simulink model "SF045A_HwAgSysArbn"  (R2013b)
settings: Solver=FixedStepDiscrete  SolverMode=SingleTasking  StartTime=0.0  StopTime=1  FixedStep=.002  RelTol=1e-3
values from neighbouring files (symbols this model uses):
  ARCHGLBPRM_2MILLISEC_SEC_F32 = DataDict.Constant    [SF045A_HwAgSysArbn_DataDict.m]
  ARCHGLBPRM_FLOATZEROTHD_ULS_F32 = DataDict.Constant    [SF045A_HwAgSysArbn_DataDict.m]
  ARCHGLBPRM_PIOVER180_ULS_F32 = DataDict.Constant    [SF045A_HwAgSysArbn_DataDict.m]
  CNVSECTOCNT_ULS_U32 = DataDict.Constant    [SF045A_HwAgSysArbn_DataDict.m]
  CNVTOMILLISEC_MILLISECPERCNT_F32 = DataDict.Constant    [SF045A_HwAgSysArbn_DataDict.m]
  FltInj_f32 = DataDict.Client    [SF045A_HwAgSysArbn_DataDict.m]
  FLTINJ_HWAGSYSARBN_HWAG = DataDict.Constant    [SF045A_HwAgSysArbn_DataDict.m]
  FLTINJ_HWAGSYSARBN_SERLCOMHWAG = DataDict.Constant    [SF045A_HwAgSysArbn_DataDict.m]
  HwAgCorrlnFlt = DataDict.NTC    [SF045A_HwAgSysArbn_DataDict.m]
  HwAgSnsrlsThdExcdd = DataDict.NTC    [SF045A_HwAgSysArbn_DataDict.m]
  HwAgSysArbnHwAgConf1Snsr = DataDict.Calibration    [SF045A_HwAgSysArbn_DataDict.m]
  HwAgSysArbnHwAgConf2Snsr = DataDict.Calibration    [SF045A_HwAgSysArbn_DataDict.m]
  HwAgSysArbnHwAgConfNoSnsr = DataDict.Calibration    [SF045A_HwAgSysArbn_DataDict.m]
  HwAgSysArbnHwAgCorrdCorrlnThd = DataDict.Calibration    [SF045A_HwAgSysArbn_DataDict.m]
  HwAgSysArbnHwAgCorrlnFailDebStep = DataDict.Calibration    [SF045A_HwAgSysArbn_DataDict.m]
  HwAgSysArbnHwAgCorrlnPassDebStep = DataDict.Calibration    [SF045A_HwAgSysArbn_DataDict.m]
  HwAgSysArbnHwAgCorrlnRng = DataDict.Calibration    [SF045A_HwAgSysArbn_DataDict.m]
  HwAgSysArbnHwAgSlewRate = DataDict.Calibration    [SF045A_HwAgSysArbn_DataDict.m]
  HwAgSysArbnHwAgSnsrlsCorrlnThd = DataDict.Calibration    [SF045A_HwAgSysArbn_DataDict.m]
  HwAgSysArbnHwAgSnsrlsKineThd = DataDict.Calibration    [SF045A_HwAgSysArbn_DataDict.m]
  HwAgSysArbnHwAgToMotAgCorrlnElpdTiLim = DataDict.Calibration    [SF045A_HwAgSysArbn_DataDict.m]
  HwAgSysArbnSerlComHwAgCorrdConf = DataDict.Calibration    [SF045A_HwAgSysArbn_DataDict.m]
  HwAgSysArbnSerlComHwAgSnsrlsConf = DataDict.Calibration    [SF045A_HwAgSysArbn_DataDict.m]
  HwAgSysArbnSlewRateTmr = DataDict.Calibration    [SF045A_HwAgSysArbn_DataDict.m]
  HWAGTHD_ULS_FLOAT32 = DataDict.Constant    [SF045A_HwAgSysArbn_DataDict.m]
  INVLDSRC_CNT_S08 = DataDict.Constant    [SF045A_HwAgSysArbn_DataDict.m]
  LRGSLEW_HWDEGPERSEC_F32 = DataDict.Constant    [SF045A_HwAgSysArbn_DataDict.m]
  NODEBSTEP_CNT_U16 = DataDict.Constant    [SF045A_HwAgSysArbn_DataDict.m]
  SLEWINPROGS_CNT_LGC = DataDict.Constant    [SF045A_HwAgSysArbn_DataDict.m]
  SLEWNOTINPROGS_CNT_LGC = DataDict.Constant    [SF045A_HwAgSysArbn_DataDict.m]
  SNSRDATASRCSELD_CNT_S08 = DataDict.Constant    [SF045A_HwAgSysArbn_DataDict.m]
  SNSRLSDATASRCSELD_CNT_S08 = DataDict.Constant    [SF045A_HwAgSysArbn_DataDict.m]
  SysGlbPrmSysKineRat = DataDict.ImprtdCal    [SF045A_HwAgSysArbn_DataDict.m]
  SysGlbPrmTorsBarStfn = DataDict.ImprtdCal    [SF045A_HwAgSysArbn_DataDict.m]
  ZEROTMR_MILLISEC_F32 = DataDict.Constant    [SF045A_HwAgSysArbn_DataDict.m]
undefined symbols (not defined in the file or in its folder): NtcSts1
libraries: NxtrLim x11, simulink x6, NxtrAbslt x6, Fil x3, autosarlib x2
(part 3 of 6)

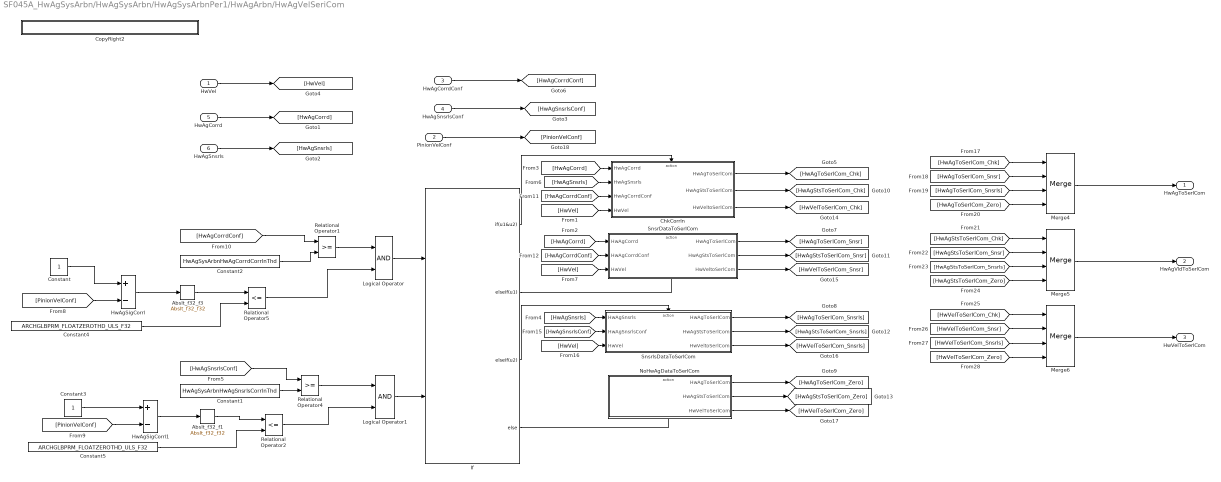
== system SF045A_HwAgSysArbn/HwAgSysArbn/HwAgSysArbnPer1/HwAgArbn/HwAgVelSeriCom ==
  HwVel : Inport
  PinionVelConf : Inport  Port=2
  HwAgCorrdConf : Inport  Port=3
  HwAgSnsrlsConf : Inport  Port=4
  HwAgCorrd : Inport  Port=5
  HwAgSnsrls : Inport  Port=6
  Abslt_f32_f1 : NxtrAbslt/Abslt_f32_f32  RequirementInfo={} %GIDa_b8a4dc3f_585f_4398_a9f9_8fc984254714  SFunctionSpec=single y1 = Abslt_f32_f32(single u1)
      settings: AttributesFormatString=%<Name>
  Abslt_f32_f3 : NxtrAbslt/Abslt_f32_f32  RequirementInfo={} %GIDa_7c7c182e_46fe_47af_9f86_60131a6a4daf  SFunctionSpec=single y1 = Abslt_f32_f32(single u1)
      settings: AttributesFormatString=%<Name>
  ChkCorrln : Subsystem  RequirementInfo="{'linktype_rmi_doors' '00012ce0 (/E-STEER Core/SubSystem Specifications/Application Functions - EA4/SF045A Handwheel Angle System Arbitration)' '#SF045A_104' 'true' 'REQ:  SF045A_104' '' ; 'linktype_rmi_doors' '00012ce0 (/E-STEER Core/SubSystem Specifications/Application Functions - EA4/SF045A Handwheel Angle System Arbitration)' '#SF045A_105' 'true' 'REQ:  SF045A_105' '' ; 'linktype_rmi_doors' '00012ce0 (/E-STEER Core/SubSystem Specifications/Application Functions - EA4/SF045A Handwheel Angle System Arbitration)' '#SF045A_141' 'true' 'REQ:  SF045A_141' '' } %GIDa_01d8e59b_3b0f_4a53_93ac_fe398fdd2570"  TreatAsAtomicUnit=on
  Constant : Constant  OutDataTypeStr=single
      settings: AttributesFormatString=%<OutDataTypeStr>
  Constant1 : Constant  RequirementInfo={} %GIDa_66b39656_3ea7_4f1f_ba8a_04f304451550  Value=HwAgSysArbnHwAgSnsrlsCorrlnThd  OutDataTypeStr=single
  Constant2 : Constant  RequirementInfo={} %GIDa_c72f589f_146e_4a47_a32d_f0a439dbf3d4  Value=HwAgSysArbnHwAgCorrdCorrlnThd  OutDataTypeStr=single
  Constant3 : Constant  OutDataTypeStr=single
      settings: AttributesFormatString=%<OutDataTypeStr>
  Constant4 : Constant  RequirementInfo={} %GIDa_2ba92f60_c072_4a0f_905b_124fe50057e6  Value=ARCHGLBPRM_FLOATZEROTHD_ULS_F32
  Constant5 : Constant  RequirementInfo={} %GIDa_95ac923c_5133_4b3b_b37a_4089be04068f  Value=ARCHGLBPRM_FLOATZEROTHD_ULS_F32
  CopyRight2 : Subsystem  Description=|  mask(Copyright Information){none=on}
      | Copyright info block.                                               
      |                                                                     
      | Place copyright information at the top of every subsystem in design.
      mask prompts: none "No parameters"
      mask help: Place copyright information at the top of every subsystem in design.
      mask Display:
      | NxtrConf = 'Nexteer Confidential';
      | 
      | sys = bdroot; %handle for the current model ("system")
      | first = get_param(sys,'Created');
      | first = first(end-3:end);  %year is last four digits
      | 
      | last = get_param(sys,'LastModifiedDate');
      | if isempty(last)
      |     last = datestr(now,'yyyy');
      | else
      |     last = last(end-3:end);
      | end
      | 
      | if strcmp(first,last)
      |     fprintf('%s -- Copyright %s Nexteer',NxtrConf,first)
      | else
      |     fprintf('%s -- %s%s- %s Nexteer',NxtrConf,char(169),first,last)
      | end
  HwAgSigCorrl : Sum  RequirementInfo="{'linktype_rmi_doors' '00012ce0 (/E-STEER Core/SubSystem Specifications/Application Functions - EA4/SF045A Handwheel Angle System Arbitration)' '#SF045A_105' 'true' 'REQ:  SF045A_105' '' } %GIDa_d7192d38_61ab_4c5a_8ed7_a2ef9f470f72"  Inputs=+-
  HwAgSigCorrl1 : Sum  RequirementInfo="{'linktype_rmi_doors' '00012ce0 (/E-STEER Core/SubSystem Specifications/Application Functions - EA4/SF045A Handwheel Angle System Arbitration)' '#SF045A_105' 'true' 'REQ:  SF045A_105' '' } %GIDa_e3eac1c3_2ea3_4330_ab07_f70996d04291"  Inputs=+-
  If : If  RequirementInfo="{'linktype_rmi_doors' '00012ce0 (/E-STEER Core/SubSystem Specifications/Application Functions - EA4/SF045A Handwheel Angle System Arbitration)' '#SF045A_85' 'true' 'REQ:  SF045A_85' '' ; 'linktype_rmi_doors' '00012ce0 (/E-STEER Core/SubSystem Specifications/Application Functions - EA4/SF045A Handwheel Angle System Arbitration)' '#SF045A_86' 'true' 'REQ:  SF045A_86' '' ; 'linktype_rmi_doors' '00012ce0 (/E-STEER Core/SubSystem Specifications/Application Functions - EA4/SF045A Handwheel Angle System Arbitration)' '#SF045A_90' 'true' 'REQ:  SF045A_90' '' ; 'linktype_rmi_doors' '00012ce0 (/E-STEER Core/SubSystem Specifications/Application Functions - EA4/SF045A Handwheel Angle System Arbitration)' '#SF045A_141' 'true' 'REQ:  SF045A_141' '' } %GIDa_16295e6d_604c_4ea2_8003_45c4a31ea523"  NumInputs=2  IfExpression=u1&u2  ElseIfExpressions=u1, u2
  Logical Operator : Logic  RequirementInfo="{'linktype_rmi_doors' '00012ce0 (/E-STEER Core/SubSystem Specifications/Application Functions - EA4/SF045A Handwheel Angle System Arbitration)' '#SF045A_104' 'true' 'REQ:  SF045A_104' '' ; 'linktype_rmi_doors' '00012ce0 (/E-STEER Core/SubSystem Specifications/Application Functions - EA4/SF045A Handwheel Angle System Arbitration)' '#SF045A_85' 'true' 'REQ:  SF045A_85' '' } %GIDa_dce261ed_e3ab_4b88_85ed_bb93f578dcbd"  AllPortsSameDT=off  OutDataTypeStr=boolean
  Logical Operator1 : Logic  RequirementInfo="{'linktype_rmi_doors' '00012ce0 (/E-STEER Core/SubSystem Specifications/Application Functions - EA4/SF045A Handwheel Angle System Arbitration)' '#SF045A_104' 'true' 'REQ:  SF045A_104' '' ; 'linktype_rmi_doors' '00012ce0 (/E-STEER Core/SubSystem Specifications/Application Functions - EA4/SF045A Handwheel Angle System Arbitration)' '#SF045A_86' 'true' 'REQ:  SF045A_86' '' } %GIDa_f647724d_ceef_4875_8752_3049c96c44e3"  AllPortsSameDT=off  OutDataTypeStr=boolean
  Merge4 : Merge  RequirementInfo="{'linktype_rmi_doors' '00012ce0 (/E-STEER Core/SubSystem Specifications/Application Functions - EA4/SF045A Handwheel Angle System Arbitration)' '#SF045A_85' 'true' 'REQ:  SF045A_85' '' ; 'linktype_rmi_doors' '00012ce0 (/E-STEER Core/SubSystem Specifications/Application Functions - EA4/SF045A Handwheel Angle System Arbitration)' '#SF045A_86' 'true' 'REQ:  SF045A_86' '' ; 'linktype_rmi_doors' '00012ce0 (/E-STEER Core/SubSystem Specifications/Application Functions - EA4/SF045A Handwheel Angle System Arbitration)' '#SF045A_141' 'true' 'REQ:  SF045A_141' '' ; 'linktype_rmi_doors' '00012ce0 (/E-STEER Core/SubSystem Specifications/Application Functions - EA4/SF045A Handwheel Angle System Arbitration)' '#SF045A_90' 'true' 'REQ:  SF045A_90' '' } %GIDa_63d2fbfa_6b1d_45be_95e0_66958795916e"  Inputs=4
  Merge5 : Merge  RequirementInfo="{'linktype_rmi_doors' '00012ce0 (/E-STEER Core/SubSystem Specifications/Application Functions - EA4/SF045A Handwheel Angle System Arbitration)' '#SF045A_85' 'true' 'REQ:  SF045A_85' '' ; 'linktype_rmi_doors' '00012ce0 (/E-STEER Core/SubSystem Specifications/Application Functions - EA4/SF045A Handwheel Angle System Arbitration)' '#SF045A_86' 'true' 'REQ:  SF045A_86' '' ; 'linktype_rmi_doors' '00012ce0 (/E-STEER Core/SubSystem Specifications/Application Functions - EA4/SF045A Handwheel Angle System Arbitration)' '#SF045A_141' 'true' 'REQ:  SF045A_141' '' ; 'linktype_rmi_doors' '00012ce0 (/E-STEER Core/SubSystem Specifications/Application Functions - EA4/SF045A Handwheel Angle System Arbitration)' '#SF045A_90' 'true' 'REQ:  SF045A_90' '' } %GIDa_9d75f2ca_ac61_4030_ae3e_b2f03a9d1071"  Inputs=4
  Merge6 : Merge  RequirementInfo="{'linktype_rmi_doors' '00012ce0 (/E-STEER Core/SubSystem Specifications/Application Functions - EA4/SF045A Handwheel Angle System Arbitration)' '#SF045A_85' 'true' 'REQ:  SF045A_85' '' ; 'linktype_rmi_doors' '00012ce0 (/E-STEER Core/SubSystem Specifications/Application Functions - EA4/SF045A Handwheel Angle System Arbitration)' '#SF045A_86' 'true' 'REQ:  SF045A_86' '' ; 'linktype_rmi_doors' '00012ce0 (/E-STEER Core/SubSystem Specifications/Application Functions - EA4/SF045A Handwheel Angle System Arbitration)' '#SF045A_141' 'true' 'REQ:  SF045A_141' '' ; 'linktype_rmi_doors' '00012ce0 (/E-STEER Core/SubSystem Specifications/Application Functions - EA4/SF045A Handwheel Angle System Arbitration)' '#SF045A_90' 'true' 'REQ:  SF045A_90' '' } %GIDa_8dbea807_2d0b_4205_9136_c887d8e00053"  Inputs=4
  NoHwAgDataToSerlCom : Subsystem  RequirementInfo="{'linktype_rmi_doors' '00012ce0 (/E-STEER Core/SubSystem Specifications/Application Functions - EA4/SF045A Handwheel Angle System Arbitration)' '#SF045A_90' 'true' 'REQ:  SF045A_90' '' } %GIDa_e15506f9_dc76_46a3_abc9_05bc78f3206f"  TreatAsAtomicUnit=on
  Relational Operator1 : RelationalOperator  RequirementInfo="{'linktype_rmi_doors' '00012ce0 (/E-STEER Core/SubSystem Specifications/Application Functions - EA4/SF045A Handwheel Angle System Arbitration)' '#SF045A_104' 'true' 'REQ:  SF045A_104' '' ; 'linktype_rmi_doors' '00012ce0 (/E-STEER Core/SubSystem Specifications/Application Functions - EA4/SF045A Handwheel Angle System Arbitration)' '#SF045A_85' 'true' 'REQ:  SF045A_85' '' } %GIDa_a51aeb99_538c_4fd9_86fe_31ab29bb7151"  OutDataTypeStr=boolean
  Relational Operator2 : RelationalOperator  RequirementInfo="{'linktype_rmi_doors' '00012ce0 (/E-STEER Core/SubSystem Specifications/Application Functions - EA4/SF045A Handwheel Angle System Arbitration)' '#SF045A_104' 'true' 'REQ:  SF045A_104' '' ; 'linktype_rmi_doors' '00012ce0 (/E-STEER Core/SubSystem Specifications/Application Functions - EA4/SF045A Handwheel Angle System Arbitration)' '#SF045A_85' 'true' 'REQ:  SF045A_85' '' } %GIDa_fbe37bb0_44f1_4683_abd9_0356a5e60375"  Operator=<=  OutDataTypeStr=boolean
  Relational Operator4 : RelationalOperator  RequirementInfo="{'linktype_rmi_doors' '00012ce0 (/E-STEER Core/SubSystem Specifications/Application Functions - EA4/SF045A Handwheel Angle System Arbitration)' '#SF045A_104' 'true' 'REQ:  SF045A_104' '' ; 'linktype_rmi_doors' '00012ce0 (/E-STEER Core/SubSystem Specifications/Application Functions - EA4/SF045A Handwheel Angle System Arbitration)' '#SF045A_86' 'true' 'REQ:  SF045A_86' '' } %GIDa_5ff63e87_12bf_4da7_987b_69d09a6b50ad"  OutDataTypeStr=boolean
  Relational Operator5 : RelationalOperator  RequirementInfo="{'linktype_rmi_doors' '00012ce0 (/E-STEER Core/SubSystem Specifications/Application Functions - EA4/SF045A Handwheel Angle System Arbitration)' '#SF045A_104' 'true' 'REQ:  SF045A_104' '' ; 'linktype_rmi_doors' '00012ce0 (/E-STEER Core/SubSystem Specifications/Application Functions - EA4/SF045A Handwheel Angle System Arbitration)' '#SF045A_85' 'true' 'REQ:  SF045A_85' '' } %GIDa_f786c2da_ebce_4ccd_8e6f_5c0e8e3ac68c"  Operator=<=  OutDataTypeStr=boolean
  SnsrDataToSerlCom : Subsystem  RequirementInfo="{'linktype_rmi_doors' '00012ce0 (/E-STEER Core/SubSystem Specifications/Application Functions - EA4/SF045A Handwheel Angle System Arbitration)' '#SF045A_85' 'true' 'REQ:  SF045A_85' '' } %GIDa_75d9779f_c388_4d50_b433_ec26c71a85aa"  TreatAsAtomicUnit=on
  SnsrlsDataToSerlCom : Subsystem  RequirementInfo="{'linktype_rmi_doors' '00012ce0 (/E-STEER Core/SubSystem Specifications/Application Functions - EA4/SF045A Handwheel Angle System Arbitration)' '#SF045A_86' 'true' 'REQ:  SF045A_86' '' ; 'linktype_rmi_doors' '00012ce0 (/E-STEER Core/SubSystem Specifications/Application Functions - EA4/SF045A Handwheel Angle System Arbitration)' '#SF045A_126' 'true' 'REQ:  SF045A_126' '' ; 'linktype_rmi_doors' '00012ce0 (/E-STEER Core/SubSystem Specifications/Application Functions - EA4/SF045A Handwheel Angle System Arbitration)' '#SF045A_124' 'true' 'REQ:  SF045A_124' '' ; 'linktype_rmi_doors' '00012ce0 (/E-STEER Core/SubSystem Specifications/Application Functions - EA4/SF045A Handwheel Angle System Arbitration)' '#SF045A_88' 'true' 'REQ:  SF045A_88' '' } %GIDa_d8bafae9_7cb5_4a99_9cbb_12d18e69b352"  TreatAsAtomicUnit=on
  HwAgToSerlCom : Outport
  HwAgVldToSerlCom : Outport  Port=2
  HwVelToSerlCom : Outport  Port=3
  wires:
  [HwAgSnsrls] -> ChkCorrln/2(HwAgSnsrls)
  [HwAgCorrdConf] -> Relational Operator1/1
  Constant2/1 -> Relational Operator1/2
  [HwAgSnsrlsConf] -> Relational Operator4/1
  Constant1/1 -> Relational Operator4/2
  If/1 -> ChkCorrln/Action
  [HwAgCorrd] -> ChkCorrln/1(HwAgCorrd)
  If/2 -> SnsrDataToSerlCom/Action
  [HwAgCorrd] -> SnsrDataToSerlCom/1(HwAgCorrd)
  [HwAgSnsrls] -> SnsrlsDataToSerlCom/1(HwAgSnsrls)
  If/3 -> SnsrlsDataToSerlCom/Action
  If/4 -> NoHwAgDataToSerlCom/Action
  [HwAgCorrdConf] -> ChkCorrln/3(HwAgCorrdConf)
  [HwAgCorrdConf] -> SnsrDataToSerlCom/2(HwAgCorrdConf)
  [HwAgSnsrlsConf] -> SnsrlsDataToSerlCom/2(HwAgSnsrlsConf)
  Merge4/1 -> HwAgToSerlCom/1
  Relational Operator1/1 -> Logical Operator/1
  Logical Operator/1 -> If/1
  Logical Operator1/1 -> If/2
  Relational Operator4/1 -> Logical Operator1/1
  [HwVel] -> ChkCorrln/4(HwVel)
  [HwVel] -> SnsrDataToSerlCom/3(HwVel)
  [HwVel] -> SnsrlsDataToSerlCom/3(HwVel)
  ChkCorrln/1(HwAgToSerlCom) -> [HwAgToSerlCom_Chk]
  SnsrDataToSerlCom/1(HwAgToSerlCom) -> [HwAgToSerlCom_Snsr]
  SnsrlsDataToSerlCom/1(HwAgToSerlCom) -> [HwAgToSerlCom_Snsrls]
  NoHwAgDataToSerlCom/1(HwAgToSerlCom) -> [HwAgToSerlCom_Zero]
  [HwAgToSerlCom_Chk] -> Merge4/1
  [HwAgToSerlCom_Snsr] -> Merge4/2
  [HwAgToSerlCom_Snsrls] -> Merge4/3
  [HwAgToSerlCom_Zero] -> Merge4/4
  ChkCorrln/2(HwAgStsToSerlCom) -> [HwAgStsToSerlCom_Chk]
  ChkCorrln/3(HwVeltoSerlCom) -> [HwVelToSerlCom_Chk]
  SnsrDataToSerlCom/2(HwAgStsToSerlCom) -> [HwAgStsToSerlCom_Snsr]
  SnsrDataToSerlCom/3(HwVeltoSerlCom) -> [HwVelToSerlCom_Snsr]
  SnsrlsDataToSerlCom/2(HwAgStsToSerlCom) -> [HwAgStsToSerlCom_Snsrls]
  SnsrlsDataToSerlCom/3(HwVeltoSerlCom) -> [HwVelToSerlCom_Snsrls]
  NoHwAgDataToSerlCom/2(HwAgStsToSerlCom) -> [HwAgStsToSerlCom_Zero]
  NoHwAgDataToSerlCom/3(HwVelToSerlCom) -> [HwVelToSerlCom_Zero]
  [HwAgStsToSerlCom_Chk] -> Merge5/1
  [HwAgStsToSerlCom_Snsr] -> Merge5/2
  [HwAgStsToSerlCom_Snsrls] -> Merge5/3
  [HwAgStsToSerlCom_Zero] -> Merge5/4
  [HwVelToSerlCom_Chk] -> Merge6/1
  [HwVelToSerlCom_Snsr] -> Merge6/2
  [HwVelToSerlCom_Snsrls] -> Merge6/3
  [HwVelToSerlCom_Zero] -> Merge6/4
  Merge6/1 -> HwVelToSerlCom/1
  HwVel/1 -> [HwVel]
  HwAgCorrdConf/1 -> [HwAgCorrdConf]
  HwAgSnsrlsConf/1 -> [HwAgSnsrlsConf]
  HwAgCorrd/1 -> [HwAgCorrd]
  HwAgSnsrls/1 -> [HwAgSnsrls]
  Merge5/1 -> HwAgVldToSerlCom/1
  PinionVelConf/1 -> [PinionVelConf]
  HwAgSigCorrl/1 -> Abslt_f32_f3/1
  Constant4/1 -> Relational Operator5/2
  Relational Operator5/1 -> Logical Operator/2
  Constant/1 -> HwAgSigCorrl/1
  [PinionVelConf] -> HwAgSigCorrl/2
  Abslt_f32_f3/1 -> Relational Operator5/1
  HwAgSigCorrl1/1 -> Abslt_f32_f1/1
  Constant5/1 -> Relational Operator2/2
  Constant3/1 -> HwAgSigCorrl1/1
  [PinionVelConf] -> HwAgSigCorrl1/2
  Abslt_f32_f1/1 -> Relational Operator2/1
  Relational Operator2/1 -> Logical Operator1/2

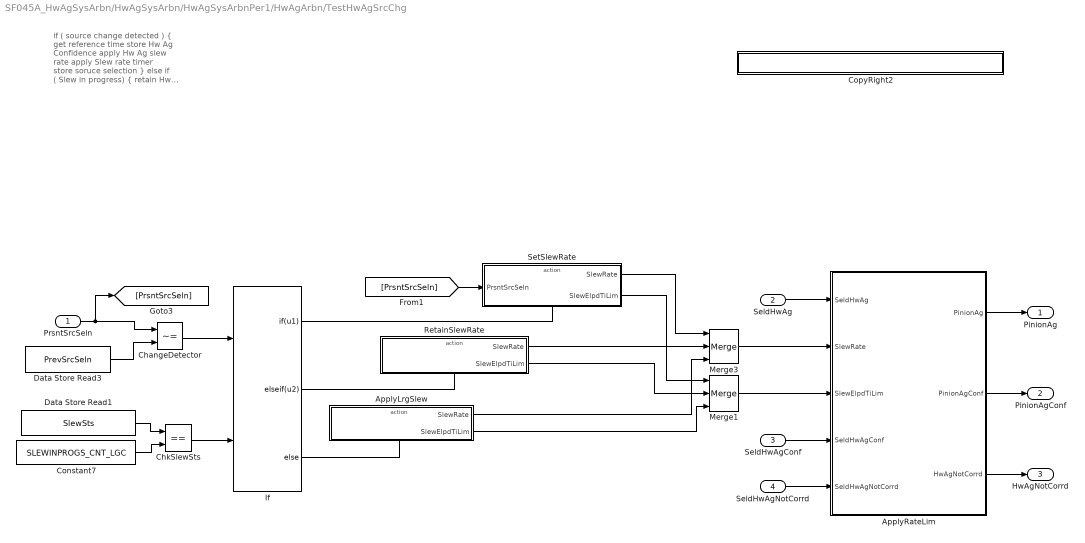
== system SF045A_HwAgSysArbn/HwAgSysArbn/HwAgSysArbnPer1/HwAgArbn/TestHwAgSrcChg ==
  note: if ( source change detected )
      | 	{
      |       get reference time
      |       store Hw Ag Confidence
      |       apply Hw Ag slew rate
      |       apply Slew rate timer
      |       store soruce selection
      | 	 }
      | else if ( Slew in progress)
      |      {
      |       retain Hw Ag slew rate
      |       retain Slew rate timer
      |       }
      |  else
      |    {
      |      apply large slew rate
      |      apply zero timer
      |     }
  PrsntSrcSeln : Inport
  SeldHwAg : Inport  Port=2
  SeldHwAgConf : Inport  Port=3
  SeldHwAgNotCorrd : Inport  Port=4
  ApplyLrgSlew : Subsystem  RequirementInfo="{'linktype_rmi_doors' '00012ce0 (/E-STEER Core/SubSystem Specifications/Application Functions - EA4/SF045A Handwheel Angle System Arbitration)' '#SF045A_77' 'true' 'REQ:  SF045A_77' '' ; 'linktype_rmi_doors' '00012ce0 (/E-STEER Core/SubSystem Specifications/Application Functions - EA4/SF045A Handwheel Angle System Arbitration)' '#SF045A_78' 'true' 'REQ:  SF045A_78' '' ; 'linktype_rmi_doors' '00012ce0 (/E-STEER Core/SubSystem Specifications/Application Functions - EA4/SF045A Handwheel Angle System Arbitration)' '#SF045A_79' 'true' 'REQ:  SF045A_79' '' } %GIDa_e44356f8_ec38_43bf_a50a_7696017339bb"  TreatAsAtomicUnit=on
  ApplyRateLim : Subsystem  RequirementInfo="{'linktype_rmi_doors' '00012ce0 (/E-STEER Core/SubSystem Specifications/Application Functions - EA4/SF045A Handwheel Angle System Arbitration)' '#SF045A_77' 'true' 'REQ:  SF045A_77' '' ; 'linktype_rmi_doors' '00012ce0 (/E-STEER Core/SubSystem Specifications/Application Functions - EA4/SF045A Handwheel Angle System Arbitration)' '#SF045A_78' 'true' 'REQ:  SF045A_78' '' ; 'linktype_rmi_doors' '00012ce0 (/E-STEER Core/SubSystem Specifications/Application Functions - EA4/SF045A Handwheel Angle System Arbitration)' '#SF045A_79' 'true' 'REQ:  SF045A_79' '' } %GIDa_f1478672_2f89_4aac_bacc_fec9bee029da"
  ChangeDetector : RelationalOperator  RequirementInfo="{'linktype_rmi_doors' '00012ce0 (/E-STEER Core/SubSystem Specifications/Application Functions - EA4/SF045A Handwheel Angle System Arbitration)' '#SF045A_77' 'true' 'REQ:  SF045A_77' '' ; 'linktype_rmi_doors' '00012ce0 (/E-STEER Core/SubSystem Specifications/Application Functions - EA4/SF045A Handwheel Angle System Arbitration)' '#SF045A_78' 'true' 'REQ:  SF045A_78' '' ; 'linktype_rmi_doors' '00012ce0 (/E-STEER Core/SubSystem Specifications/Application Functions - EA4/SF045A Handwheel Angle System Arbitration)' '#SF045A_79' 'true' 'REQ:  SF045A_79' '' } %GIDa_8b7e8362_f8ac_4ce7_bdd9_53ebc347e7a4"  Operator=~=  OutDataTypeStr=boolean
  ChkSlewSts : RelationalOperator  RequirementInfo="{'linktype_rmi_doors' '00012ce0 (/E-STEER Core/SubSystem Specifications/Application Functions - EA4/SF045A Handwheel Angle System Arbitration)' '#SF045A_77' 'true' 'REQ:  SF045A_77' '' ; 'linktype_rmi_doors' '00012ce0 (/E-STEER Core/SubSystem Specifications/Application Functions - EA4/SF045A Handwheel Angle System Arbitration)' '#SF045A_78' 'true' 'REQ:  SF045A_78' '' ; 'linktype_rmi_doors' '00012ce0 (/E-STEER Core/SubSystem Specifications/Application Functions - EA4/SF045A Handwheel Angle System Arbitration)' '#SF045A_79' 'true' 'REQ:  SF045A_79' '' } %GIDa_bfec169c_9d41_4bc2_ac68_6c555ee4a7f9"  Operator===  OutDataTypeStr=boolean
  Constant7 : Constant  Value=SLEWINPROGS_CNT_LGC
  CopyRight2 : Subsystem  Description=|  mask(Copyright Information){none=on}
      | Copyright info block.                                               
      |                                                                     
      | Place copyright information at the top of every subsystem in design.
      mask prompts: none "No parameters"
      mask help: Place copyright information at the top of every subsystem in design.
      mask Display:
      | NxtrConf = 'Nexteer Confidential';
      | 
      | sys = bdroot; %handle for the current model ("system")
      | first = get_param(sys,'Created');
      | first = first(end-3:end);  %year is last four digits
      | 
      | last = get_param(sys,'LastModifiedDate');
      | if isempty(last)
      |     last = datestr(now,'yyyy');
      | else
      |     last = last(end-3:end);
      | end
      | 
      | if strcmp(first,last)
      |     fprintf('%s -- Copyright %s Nexteer',NxtrConf,first)
      | else
      |     fprintf('%s -- %s%s- %s Nexteer',NxtrConf,char(169),first,last)
      | end
  Data Store Read1 : DataStoreRead  RequirementInfo="{'linktype_rmi_doors' '00012ce0 (/E-STEER Core/SubSystem Specifications/Application Functions - EA4/SF045A Handwheel Angle System Arbitration)' '#SF045A_77' 'true' 'REQ:  SF045A_77' '' } %GIDa_50bb0bd0_a46e_4acc_84f3_31f30c152d08"  DataStoreName=SlewSts
  Data Store Read3 : DataStoreRead  RequirementInfo={} %GIDa_1f3832b3_ed57_4269_9832_05f59754d85e  DataStoreName=PrevSrcSeln
  If : If  RequirementInfo="{'linktype_rmi_doors' '00012ce0 (/E-STEER Core/SubSystem Specifications/Application Functions - EA4/SF045A Handwheel Angle System Arbitration)' '#SF045A_77' 'true' 'REQ:  SF045A_77' '' } %GIDa_3988356c_2296_425a_9b51_6ae96000ad4c"  NumInputs=2  IfExpression=u1  ElseIfExpressions=u2
  Merge1 : Merge  RequirementInfo="{'linktype_rmi_doors' '00012ce0 (/E-STEER Core/SubSystem Specifications/Application Functions - EA4/SF045A Handwheel Angle System Arbitration)' '#SF045A_77' 'true' 'REQ:  SF045A_77' '' ; 'linktype_rmi_doors' '00012ce0 (/E-STEER Core/SubSystem Specifications/Application Functions - EA4/SF045A Handwheel Angle System Arbitration)' '#SF045A_78' 'true' 'REQ:  SF045A_78' '' ; 'linktype_rmi_doors' '00012ce0 (/E-STEER Core/SubSystem Specifications/Application Functions - EA4/SF045A Handwheel Angle System Arbitration)' '#SF045A_79' 'true' 'REQ:  SF045A_79' '' } %GIDa_d9ff7edc_00ec_4746_8c06_dd030c724f9b"  Inputs=3
  Merge3 : Merge  RequirementInfo="{'linktype_rmi_doors' '00012ce0 (/E-STEER Core/SubSystem Specifications/Application Functions - EA4/SF045A Handwheel Angle System Arbitration)' '#SF045A_77' 'true' 'REQ:  SF045A_77' '' ; 'linktype_rmi_doors' '00012ce0 (/E-STEER Core/SubSystem Specifications/Application Functions - EA4/SF045A Handwheel Angle System Arbitration)' '#SF045A_78' 'true' 'REQ:  SF045A_78' '' ; 'linktype_rmi_doors' '00012ce0 (/E-STEER Core/SubSystem Specifications/Application Functions - EA4/SF045A Handwheel Angle System Arbitration)' '#SF045A_79' 'true' 'REQ:  SF045A_79' '' } %GIDa_987ee040_1718_40a9_8501_c39e0ec1e0d7"  Inputs=3
  RetainSlewRate : Subsystem  RequirementInfo="{'linktype_rmi_doors' '00012ce0 (/E-STEER Core/SubSystem Specifications/Application Functions - EA4/SF045A Handwheel Angle System Arbitration)' '#SF045A_77' 'true' 'REQ:  SF045A_77' '' ; 'linktype_rmi_doors' '00012ce0 (/E-STEER Core/SubSystem Specifications/Application Functions - EA4/SF045A Handwheel Angle System Arbitration)' '#SF045A_78' 'true' 'REQ:  SF045A_78' '' ; 'linktype_rmi_doors' '00012ce0 (/E-STEER Core/SubSystem Specifications/Application Functions - EA4/SF045A Handwheel Angle System Arbitration)' '#SF045A_79' 'true' 'REQ:  SF045A_79' '' } %GIDa_4bf0b3c8_ee1f_4198_a4a1_a06a6fb30b87"  TreatAsAtomicUnit=on
  SetSlewRate : Subsystem  RequirementInfo="{'linktype_rmi_doors' '00012ce0 (/E-STEER Core/SubSystem Specifications/Application Functions - EA4/SF045A Handwheel Angle System Arbitration)' '#SF045A_77' 'true' 'REQ:  SF045A_77' '' ; 'linktype_rmi_doors' '00012ce0 (/E-STEER Core/SubSystem Specifications/Application Functions - EA4/SF045A Handwheel Angle System Arbitration)' '#SF045A_78' 'true' 'REQ:  SF045A_78' '' ; 'linktype_rmi_doors' '00012ce0 (/E-STEER Core/SubSystem Specifications/Application Functions - EA4/SF045A Handwheel Angle System Arbitration)' '#SF045A_79' 'true' 'REQ:  SF045A_79' '' } %GIDa_5f10b8d5_5a39_4d87_9d6f_026f32a004c2"  TreatAsAtomicUnit=on
  PinionAg : Outport
  PinionAgConf : Outport  Port=2
  HwAgNotCorrd : Outport  Port=3
  wires:
  If/3 -> ApplyLrgSlew/Action
  SeldHwAg/1 -> ApplyRateLim/1(SeldHwAg)
  Merge3/1 -> ApplyRateLim/2(SlewRate)
  Merge1/1 -> ApplyRateLim/3(SlewElpdTiLim)
  ApplyRateLim/2(PinionAgConf) -> PinionAgConf/1
  ApplyRateLim/3(HwAgNotCorrd) -> HwAgNotCorrd/1
  ApplyRateLim/1(PinionAg) -> PinionAg/1
  SeldHwAgConf/1 -> ApplyRateLim/4(SeldHwAgConf)
  SeldHwAgNotCorrd/1 -> ApplyRateLim/5(SeldHwAgNotCorrd)
  If/1 -> SetSlewRate/Action
  If/2 -> RetainSlewRate/Action
  PrsntSrcSeln/1 -> ChangeDetector/1, [PrsntSrcSeln]
  Data Store Read3/1 -> ChangeDetector/2
  ChangeDetector/1 -> If/1
  [PrsntSrcSeln] -> SetSlewRate/1(PrsntSrcSeln)
  Data Store Read1/1 -> ChkSlewSts/1
  Constant7/1 -> ChkSlewSts/2
  ChkSlewSts/1 -> If/2
  SetSlewRate/1(SlewRate) -> Merge3/1
  RetainSlewRate/1(SlewRate) -> Merge3/2
  ApplyLrgSlew/2(SlewElpdTiLim) -> Merge1/3
  ApplyLrgSlew/1(SlewRate) -> Merge3/3
  SetSlewRate/2("SlewElpdTiLim ") -> Merge1/1
  RetainSlewRate/2("SlewElpdTiLim ") -> Merge1/2

== system SF045A_HwAgSysArbn/HwAgSysArbn/HwAgSysArbnPer1/HwAgArbn/VldtSnsrlsData ==
  HwAgSnsrlsIn : Inport
  HwAgSnsrlsConfIn : Inport  Port=2
  Abslt_f32_f1 : NxtrAbslt/Abslt_f32_f32  RequirementInfo="{'linktype_rmi_doors' '00012ce0 (/E-STEER Core/SubSystem Specifications/Application Functions - EA4/SF045A Handwheel Angle System Arbitration)' '#SF045A_69' 'true' 'REQ:  SF045A_69' '' } %GIDa_11557de6_db47_45ed_8bfc_c441158f19d2"  SFunctionSpec=single y1 = Abslt_f32_f32(single u1)
      settings: AttributesFormatString=%<Name>
  Constant7 : Constant  RequirementInfo={} %GIDa_38fba33f_478a_4437_a0d9_970a62fe73dd  Value=HwAgSysArbnHwAgSnsrlsKineThd
  CopyRight2 : Subsystem  Description=|  mask(Copyright Information){none=on}
      | Copyright info block.                                               
      |                                                                     
      | Place copyright information at the top of every subsystem in design.
      mask prompts: none "No parameters"
      mask help: Place copyright information at the top of every subsystem in design.
      mask Display:
      | NxtrConf = 'Nexteer Confidential';
      | 
      | sys = bdroot; %handle for the current model ("system")
      | first = get_param(sys,'Created');
      | first = first(end-3:end);  %year is last four digits
      | 
      | last = get_param(sys,'LastModifiedDate');
      | if isempty(last)
      |     last = datestr(now,'yyyy');
      | else
      |     last = last(end-3:end);
      | end
      | 
      | if strcmp(first,last)
      |     fprintf('%s -- Copyright %s Nexteer',NxtrConf,first)
      | else
      |     fprintf('%s -- %s%s- %s Nexteer',NxtrConf,char(169),first,last)
      | end
  Data Store Read2 : DataStoreRead  RequirementInfo="{'linktype_rmi_doors' '00012ce0 (/E-STEER Core/SubSystem Specifications/Application Functions - EA4/SF045A Handwheel Angle System Arbitration)' '#SF045A_69' 'true' 'REQ:  SF045A_69' '' } %GIDa_3297d32f_1510_4b0f_8fc3_e93c18620b92"  DataStoreName=HwAgKineFlt
  If : If  RequirementInfo="{'linktype_rmi_doors' '00012ce0 (/E-STEER Core/SubSystem Specifications/Application Functions - EA4/SF045A Handwheel Angle System Arbitration)' '#SF045A_69' 'true' 'REQ:  SF045A_69' '' } %GIDa_2be10aed_c199_4185_9877_aa6fe9b11c28"  IfExpression=u1
  Logical Operator : Logic  RequirementInfo="{'linktype_rmi_doors' '00012ce0 (/E-STEER Core/SubSystem Specifications/Application Functions - EA4/SF045A Handwheel Angle System Arbitration)' '#SF045A_69' 'true' 'REQ:  SF045A_69' '' } %GIDa_d3f639fb_b632_4a47_9a92_53825d00e1fa"  Operator=NOT  AllPortsSameDT=off  OutDataTypeStr=boolean
  Logical Operator1 : Logic  RequirementInfo="{'linktype_rmi_doors' '00012ce0 (/E-STEER Core/SubSystem Specifications/Application Functions - EA4/SF045A Handwheel Angle System Arbitration)' '#SF045A_69' 'true' 'REQ:  SF045A_69' '' } %GIDa_5b8fbd5c_2375_4aab_90b1_9acca4547e18"  AllPortsSameDT=off  OutDataTypeStr=boolean
  Merge1 : Merge  RequirementInfo="{'linktype_rmi_doors' '00012ce0 (/E-STEER Core/SubSystem Specifications/Application Functions - EA4/SF045A Handwheel Angle System Arbitration)' '#SF045A_69' 'true' 'REQ:  SF045A_69' '' } %GIDa_f2974614_a6c0_4132_871a_85df54ea8bdb"
  Pass : Subsystem  RequirementInfo="{'linktype_rmi_doors' '00012ce0 (/E-STEER Core/SubSystem Specifications/Application Functions - EA4/SF045A Handwheel Angle System Arbitration)' '#SF045A_69' 'true' 'REQ:  SF045A_69' '' } %GIDa_40ca0eea_dda3_4113_aa3b_c2f7ee942c93"  TreatAsAtomicUnit=on
  Relational Operator4 : RelationalOperator  RequirementInfo="{'linktype_rmi_doors' '00012ce0 (/E-STEER Core/SubSystem Specifications/Application Functions - EA4/SF045A Handwheel Angle System Arbitration)' '#SF045A_69' 'true' 'REQ:  SF045A_69' '' } %GIDa_7a726458_a836_43ae_989d_bcf3c6c47486"  Operator=<=  OutDataTypeStr=boolean
  ThdExcdd : Subsystem  RequirementInfo="{'linktype_rmi_doors' '00012ce0 (/E-STEER Core/SubSystem Specifications/Application Functions - EA4/SF045A Handwheel Angle System Arbitration)' '#SF045A_69' 'true' 'REQ:  SF045A_69' '' ; 'linktype_rmi_doors' '00012ce0 (/E-STEER Core/SubSystem Specifications/Application Functions - EA4/SF045A Handwheel Angle System Arbitration)' '#SF045A_95' 'true' 'REQ:  SF045A_95' '' ; 'linktype_rmi_doors' '00012ce0 (/E-STEER Core/SubSystem Specifications/Application Functions - EA4/SF045A Handwheel Angle System Arbitration)' '#SF045A_114' 'true' 'REQ:  SF045A_114' '' } %GIDa_388bca23_10d4_4a82_9a17_1d57e5c6edc8"  TreatAsAtomicUnit=on
  HwAgSnsrlsConf : Outport
  wires:
  Abslt_f32_f1/1 -> Relational Operator4/1
  ThdExcdd/1(Out) -> Merge1/2
  HwAgSnsrlsIn/1 -> Abslt_f32_f1/1
  Constant7/1 -> Relational Operator4/2
  If/1 -> Pass/Action
  If/2 -> ThdExcdd/Action
  Merge1/1 -> HwAgSnsrlsConf/1
  HwAgSnsrlsConfIn/1 -> Pass/1(In)
  Relational Operator4/1 -> Logical Operator1/1
  Data Store Read2/1 -> Logical Operator/1
  Logical Operator/1 -> Logical Operator1/2
  Logical Operator1/1 -> If/1
  Pass/1(Out) -> Merge1/1

== system SF045A_HwAgSysArbn/HwAgSysArbn/HwAgSysArbnInit1/Kinematic Integrity/SetNtcSts/CopyRight2 ==

== system SF045A_HwAgSysArbn/HwAgSysArbn/HwAgSysArbnPer1/FltInj_f32 client/CodeGen/CopyRight1 ==

== system SF045A_HwAgSysArbn/HwAgSysArbn/HwAgSysArbnPer1/FltInj_f32 client/Sim/CopyRight1 ==

== system SF045A_HwAgSysArbn/HwAgSysArbn/HwAgSysArbnPer1/FltInj_f32 client1/CodeGen/CopyRight1 ==

== system SF045A_HwAgSysArbn/HwAgSysArbn/HwAgSysArbnPer1/FltInj_f32 client1/Sim/CopyRight1 ==

== system SF045A_HwAgSysArbn/HwAgSysArbn/HwAgSysArbnPer1/HwAgArbn/CalcHwAgCorrdConf /CopyRight2 ==

== system SF045A_HwAgSysArbn/HwAgSysArbn/HwAgSysArbnPer1/HwAgArbn/CalcHwAgCorrdConf /NoSensor ==
  Action Port : ActionPort  ActionType=case
  Constant6 : Constant  RequirementInfo={} %GIDa_5ce1f3ce_a703_4b49_a05d_c5b5f94c45b6  Value=HwAgSysArbnHwAgConfNoSnsr
  CopyRight2 : Subsystem  Description=|  mask(Copyright Information){none=on}
      | Copyright info block.                                               
      |                                                                     
      | Place copyright information at the top of every subsystem in design.
      mask prompts: none "No parameters"
      mask help: Place copyright information at the top of every subsystem in design.
      mask Display:
      | NxtrConf = 'Nexteer Confidential';
      | 
      | sys = bdroot; %handle for the current model ("system")
      | first = get_param(sys,'Created');
      | first = first(end-3:end);  %year is last four digits
      | 
      | last = get_param(sys,'LastModifiedDate');
      | if isempty(last)
      |     last = datestr(now,'yyyy');
      | else
      |     last = last(end-3:end);
      | end
      | 
      | if strcmp(first,last)
      |     fprintf('%s -- Copyright %s Nexteer',NxtrConf,first)
      | else
      |     fprintf('%s -- %s%s- %s Nexteer',NxtrConf,char(169),first,last)
      | end
  Out1 : Outport
  wires:
  Constant6/1 -> Out1/1

== system SF045A_HwAgSysArbn/HwAgSysArbn/HwAgSysArbnPer1/HwAgArbn/CalcHwAgCorrdConf /OneSensor ==
  Action Port : ActionPort  ActionType=case
  Constant6 : Constant  RequirementInfo={} %GIDa_53d3376b_c1a7_4d30_9373_dc2601928419  Value=HwAgSysArbnHwAgConf1Snsr
  CopyRight2 : Subsystem  Description=|  mask(Copyright Information){none=on}
      | Copyright info block.                                               
      |                                                                     
      | Place copyright information at the top of every subsystem in design.
      mask prompts: none "No parameters"
      mask help: Place copyright information at the top of every subsystem in design.
      mask Display:
      | NxtrConf = 'Nexteer Confidential';
      | 
      | sys = bdroot; %handle for the current model ("system")
      | first = get_param(sys,'Created');
      | first = first(end-3:end);  %year is last four digits
      | 
      | last = get_param(sys,'LastModifiedDate');
      | if isempty(last)
      |     last = datestr(now,'yyyy');
      | else
      |     last = last(end-3:end);
      | end
      | 
      | if strcmp(first,last)
      |     fprintf('%s -- Copyright %s Nexteer',NxtrConf,first)
      | else
      |     fprintf('%s -- %s%s- %s Nexteer',NxtrConf,char(169),first,last)
      | end
  Out1 : Outport
  wires:
  Constant6/1 -> Out1/1

== system SF045A_HwAgSysArbn/HwAgSysArbn/HwAgSysArbnPer1/HwAgArbn/CalcHwAgCorrdConf /TwoSensors ==
  Action Port : ActionPort  ActionType=case
  Constant5 : Constant  RequirementInfo={} %GIDa_145a2860_1a8e_4a78_b839_766063a3a5fa  Value=HwAgSysArbnHwAgConf2Snsr  OutDataTypeStr=single
      settings: AttributesFormatString=%<OutDataTypeStr>
  CopyRight2 : Subsystem  Description=|  mask(Copyright Information){none=on}
      | Copyright info block.                                               
      |                                                                     
      | Place copyright information at the top of every subsystem in design.
      mask prompts: none "No parameters"
      mask help: Place copyright information at the top of every subsystem in design.
      mask Display:
      | NxtrConf = 'Nexteer Confidential';
      | 
      | sys = bdroot; %handle for the current model ("system")
      | first = get_param(sys,'Created');
      | first = first(end-3:end);  %year is last four digits
      | 
      | last = get_param(sys,'LastModifiedDate');
      | if isempty(last)
      |     last = datestr(now,'yyyy');
      | else
      |     last = last(end-3:end);
      | end
      | 
      | if strcmp(first,last)
      |     fprintf('%s -- Copyright %s Nexteer',NxtrConf,first)
      | else
      |     fprintf('%s -- %s%s- %s Nexteer',NxtrConf,char(169),first,last)
      | end
  Out1 : Outport
  wires:
  Constant5/1 -> Out1/1

== system SF045A_HwAgSysArbn/HwAgSysArbn/HwAgSysArbnPer1/HwAgArbn/CalcHwAgCorrdConf /Zero ==
  Action Port : ActionPort  ActionType=default
  Constant5 : Constant  RequirementInfo={} %GIDa_61ee8135_2090_4e08_8456_cbda17ec1ca3  Value=0  OutDataTypeStr=single
      settings: AttributesFormatString=%<OutDataTypeStr>
  CopyRight2 : Subsystem  Description=|  mask(Copyright Information){none=on}
      | Copyright info block.                                               
      |                                                                     
      | Place copyright information at the top of every subsystem in design.
      mask prompts: none "No parameters"
      mask help: Place copyright information at the top of every subsystem in design.
      mask Display:
      | NxtrConf = 'Nexteer Confidential';
      | 
      | sys = bdroot; %handle for the current model ("system")
      | first = get_param(sys,'Created');
      | first = first(end-3:end);  %year is last four digits
      | 
      | last = get_param(sys,'LastModifiedDate');
      | if isempty(last)
      |     last = datestr(now,'yyyy');
      | else
      |     last = last(end-3:end);
      | end
      | 
      | if strcmp(first,last)
      |     fprintf('%s -- Copyright %s Nexteer',NxtrConf,first)
      | else
      |     fprintf('%s -- %s%s- %s Nexteer',NxtrConf,char(169),first,last)
      | end
  Out1 : Outport
  wires:
  Constant5/1 -> Out1/1

== system SF045A_HwAgSysArbn/HwAgSysArbn/HwAgSysArbnPer1/HwAgArbn/CalcPinionVel/CopyRight2 ==

== system SF045A_HwAgSysArbn/HwAgSysArbn/HwAgSysArbnPer1/HwAgArbn/CalcPinionVel/MotorVelocityVld ==
  MotVelCrf : Inport
  HwTq : Inport  RequirementInfo={} %GIDa_8ab325fa_5ec7_4465_9250_3b546f98988d  Port=2
  Action Port : ActionPort  ActionType=then
  Add : Sum  RequirementInfo="{'linktype_rmi_doors' '00012ce0 (/E-STEER Core/SubSystem Specifications/Application Functions - EA4/SF045A Handwheel Angle System Arbitration)' '#SF045A_138' 'true' 'REQ:  SF045A_138' '' } %GIDa_5304434e_1407_4649_b941_68a6623380be"
  Constant : Constant  OutDataTypeStr=single
      settings: AttributesFormatString=%<OutDataTypeStr>
  CopyRight2 : Subsystem  Description=|  mask(Copyright Information){none=on}
      | Copyright info block.                                               
      |                                                                     
      | Place copyright information at the top of every subsystem in design.
      mask prompts: none "No parameters"
      mask help: Place copyright information at the top of every subsystem in design.
      mask Display:
      | NxtrConf = 'Nexteer Confidential';
      | 
      | sys = bdroot; %handle for the current model ("system")
      | first = get_param(sys,'Created');
      | first = first(end-3:end);  %year is last four digits
      | 
      | last = get_param(sys,'LastModifiedDate');
      | if isempty(last)
      |     last = datestr(now,'yyyy');
      | else
      |     last = last(end-3:end);
      | end
      | 
      | if strcmp(first,last)
      |     fprintf('%s -- Copyright %s Nexteer',NxtrConf,first)
      | else
      |     fprintf('%s -- %s%s- %s Nexteer',NxtrConf,char(169),first,last)
      | end
  Mult2 : Product  RequirementInfo="{'linktype_rmi_doors' '00012ce0 (/E-STEER Core/SubSystem Specifications/Application Functions - EA4/SF045A Handwheel Angle System Arbitration)' '#SF045A_138' 'true' 'REQ:  SF045A_138' '' } %GIDa_fe66ac48_e0c5_4c57_b872_a36bd11fb71b"  Inputs=*/
  TbarVelocity : Subsystem  Tag=Calculate Driver Velocity  Description=Driver Velocity is pinion velocity +/- the effect of T-bar twist.  RequirementInfo="{'linktype_rmi_doors' '00012ce0 (/E-STEER Core/SubSystem Specifications/Application Functions - EA4/SF045A Handwheel Angle System Arbitration)' '#SF045A_137' 'true' 'REQ:  SF045A_137' '' } %GIDa_8e292011_d4ba_4fe9_b071_7395ab527a64"  TreatAsAtomicUnit=on
  k_Mtr2HwRatio_MtrDegpHwDeg : Constant  RequirementInfo="{'linktype_rmi_doors' '00012ce0 (/E-STEER Core/SubSystem Specifications/Application Functions - EA4/SF045A Handwheel Angle System Arbitration)' '#SF045A_138' 'true' 'REQ:  SF045A_138' '' } %GIDa_36f93249_0236_456b_9a54_26fd8d985ff2"  Value=SysGlbPrmSysKineRat
  MotVld_PinionVel : Outport
  MotVld_HwVel : Outport  Port=2
  MotVld_PinionVelConf : Outport  Port=3
  wires:
  MotVelCrf/1 -> Mult2/1
  k_Mtr2HwRatio_MtrDegpHwDeg/1 -> Mult2/2
  HwTq/1 -> TbarVelocity/1(HwTq)
  TbarVelocity/1(TbarVel) -> Add/2  "TbarVel_HwRadPerSec_T_f32"
  Mult2/1 -> Add/1, MotVld_PinionVel/1  "PinionVel_HwRadPerSec_T_f32"
  Add/1 -> MotVld_HwVel/1
  Constant/1 -> MotVld_PinionVelConf/1

== system SF045A_HwAgSysArbn/HwAgSysArbn/HwAgSysArbnPer1/HwAgArbn/CalcPinionVel/PinionAnglegConf ==
  HwTq : Inport
  HwAg : Inport  Port=2
  Action Port : ActionPort  ActionType=elseif
  Add1 : Sum  RequirementInfo="{'linktype_rmi_doors' '00012ce0 (/E-STEER Core/SubSystem Specifications/Application Functions - EA4/SF045A Handwheel Angle System Arbitration)' '#SF045A_139' 'true' 'REQ:  SF045A_139' '' } %GIDa_c6b40892_6bbb_4386_b768_13fc7c79763b"
  Constant : Constant  OutDataTypeStr=single
      settings: AttributesFormatString=%<OutDataTypeStr>
  CopyRight2 : Subsystem  Description=|  mask(Copyright Information){none=on}
      | Copyright info block.                                               
      |                                                                     
      | Place copyright information at the top of every subsystem in design.
      mask prompts: none "No parameters"
      mask help: Place copyright information at the top of every subsystem in design.
      mask Display:
      | NxtrConf = 'Nexteer Confidential';
      | 
      | sys = bdroot; %handle for the current model ("system")
      | first = get_param(sys,'Created');
      | first = first(end-3:end);  %year is last four digits
      | 
      | last = get_param(sys,'LastModifiedDate');
      | if isempty(last)
      |     last = datestr(now,'yyyy');
      | else
      |     last = last(end-3:end);
      | end
      | 
      | if strcmp(first,last)
      |     fprintf('%s -- Copyright %s Nexteer',NxtrConf,first)
      | else
      |     fprintf('%s -- %s%s- %s Nexteer',NxtrConf,char(169),first,last)
      | end
  HwAg_Derivative : Subsystem  Tag=Calculate Driver Velocity  Description=Driver Velocity is pinion velocity +/- the effect of T-bar twist.  RequirementInfo="{'linktype_rmi_doors' '00012ce0 (/E-STEER Core/SubSystem Specifications/Application Functions - EA4/SF045A Handwheel Angle System Arbitration)' '#SF045A_139' 'true' 'REQ:  SF045A_139' '' } %GIDa_e1c810ea_54be_40d5_968c_35659183f21b"  TreatAsAtomicUnit=on
  TbarVelocity : Subsystem  Tag=Calculate Driver Velocity  Description=Driver Velocity is pinion velocity +/- the effect of T-bar twist.  RequirementInfo="{'linktype_rmi_doors' '00012ce0 (/E-STEER Core/SubSystem Specifications/Application Functions - EA4/SF045A Handwheel Angle System Arbitration)' '#SF045A_137' 'true' 'REQ:  SF045A_137' '' ; 'linktype_rmi_doors' '00012ce0 (/E-STEER Core/SubSystem Specifications/Application Functions - EA4/SF045A Handwheel Angle System Arbitration)' '#SF045A_139' 'true' 'REQ:  SF045A_139' '' } %GIDa_2a0b1cfb_ae23_4a9b_af9f_ab24977cb864"  TreatAsAtomicUnit=on
  PinionAgConf_PinionVel : Outport
  PinionAgConf_HwVel : Outport  Port=2
  PinionAgConf_PinionVelConf : Outport  Port=3
  wires:
  TbarVelocity/1(TbarVel) -> Add1/2  "TbarVel_HwRadPerSec_T_f32"
  HwAg_Derivative/1(HwAg_Der) -> Add1/1, PinionAgConf_PinionVel/1  "HwAgDer_HwRadPerSec_T_f32"
  Add1/1 -> PinionAgConf_HwVel/1
  Constant/1 -> PinionAgConf_PinionVelConf/1
  HwTq/1 -> TbarVelocity/1(HwTq)
  HwAg/1 -> HwAg_Derivative/1(HwAg)

== system SF045A_HwAgSysArbn/HwAgSysArbn/HwAgSysArbnPer1/HwAgArbn/CalcPinionVel/ZeroState ==
  Action Port : ActionPort  ActionType=else
  CopyRight2 : Subsystem  Description=|  mask(Copyright Information){none=on}
      | Copyright info block.                                               
      |                                                                     
      | Place copyright information at the top of every subsystem in design.
      mask prompts: none "No parameters"
      mask help: Place copyright information at the top of every subsystem in design.
      mask Display:
      | NxtrConf = 'Nexteer Confidential';
      | 
      | sys = bdroot; %handle for the current model ("system")
      | first = get_param(sys,'Created');
      | first = first(end-3:end);  %year is last four digits
      | 
      | last = get_param(sys,'LastModifiedDate');
      | if isempty(last)
      |     last = datestr(now,'yyyy');
      | else
      |     last = last(end-3:end);
      | end
      | 
      | if strcmp(first,last)
      |     fprintf('%s -- Copyright %s Nexteer',NxtrConf,first)
      | else
      |     fprintf('%s -- %s%s- %s Nexteer',NxtrConf,char(169),first,last)
      | end
  HwVelFalse : Constant  Value=0  OutDataTypeStr=single
      settings: AttributesFormatString=%<OutDataTypeStr>
  PinionVelConfFalse : Constant  Value=0  OutDataTypeStr=single
      settings: AttributesFormatString=%<OutDataTypeStr>
  PinionVelFalse : Constant  Value=0  OutDataTypeStr=single
      settings: AttributesFormatString=%<OutDataTypeStr>
  FALSE_PinionVel : Outport
  FALSE_HwVel : Outport  Port=2
  FALSE_PinionVelConf : Outport  Port=3
  wires:
  PinionVelFalse/1 -> FALSE_PinionVel/1
  HwVelFalse/1 -> FALSE_HwVel/1
  PinionVelConfFalse/1 -> FALSE_PinionVelConf/1

== system SF045A_HwAgSysArbn/HwAgSysArbn/HwAgSysArbnPer1/HwAgArbn/HwAgSrcSeln/CopyRight2 ==

== system SF045A_HwAgSysArbn/HwAgSysArbn/HwAgSysArbnPer1/HwAgArbn/HwAgSrcSeln/SnsrlsHwAgSeln ==
  HwAgSnsrls : Inport
  HwAgSnsrlsConf : Inport  Port=2
  Action Port : ActionPort  ActionType=else
  CopyRight2 : Subsystem  Description=|  mask(Copyright Information){none=on}
      | Copyright info block.                                               
      |                                                                     
      | Place copyright information at the top of every subsystem in design.
      mask prompts: none "No parameters"
      mask help: Place copyright information at the top of every subsystem in design.
      mask Display:
      | NxtrConf = 'Nexteer Confidential';
      | 
      | sys = bdroot; %handle for the current model ("system")
      | first = get_param(sys,'Created');
      | first = first(end-3:end);  %year is last four digits
      | 
      | last = get_param(sys,'LastModifiedDate');
      | if isempty(last)
      |     last = datestr(now,'yyyy');
      | else
      |     last = last(end-3:end);
      | end
      | 
      | if strcmp(first,last)
      |     fprintf('%s -- Copyright %s Nexteer',NxtrConf,first)
      | else
      |     fprintf('%s -- %s%s- %s Nexteer',NxtrConf,char(169),first,last)
      | end
  SET : Constant  Value=SNSRLSDATASRCSELD_CNT_S08
  HwAgOut : Outport
  HwAgConfOut : Outport  Port=2
  HwAgNotCorrd : Outport  Port=3
  SrcSeln : Outport  Port=4
  wires:
  HwAgSnsrlsConf/1 -> HwAgConfOut/1
  HwAgSnsrls/1 -> HwAgNotCorrd/1, HwAgOut/1
  SET/1 -> SrcSeln/1
